simulink model "testmodel"  (R2017b)
settings: Solver=ode3  StartTime=0.0  StopTime=100  FixedStep=0.001  RelTol=1e-3
undefined symbols (not defined in the file or in its folder): DiscIntNeverNeededParam
libraries: simulink_extras x2, simulink x1
settings Model: Creator=apple  LastModifiedBy=apple
settings DebuggingCC: AlgebraicLoopMsg=none

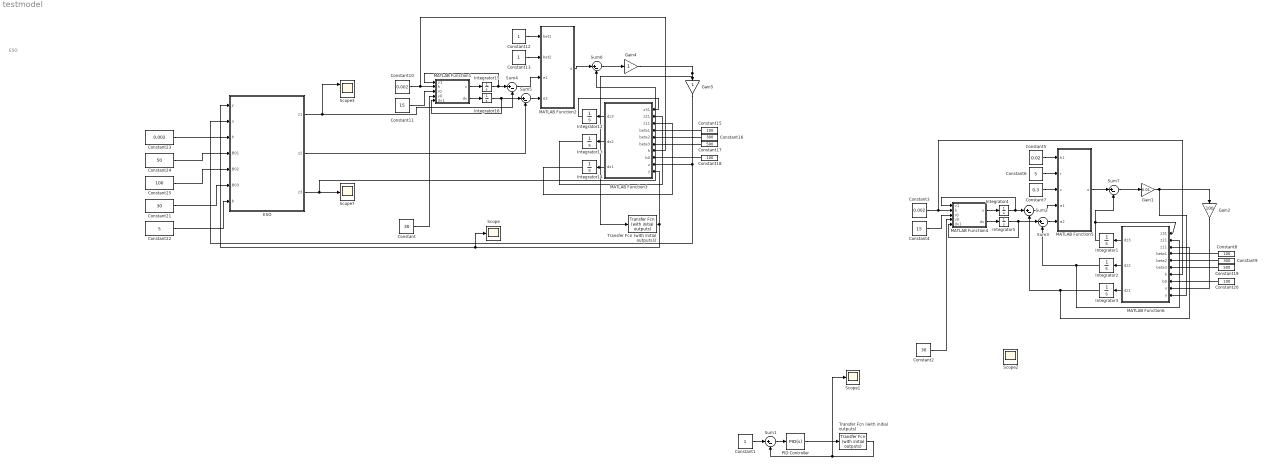
== system testmodel ==
  note: ESO
  Constant : Constant  Value=30
  Constant1 : Constant
  Constant10 : Constant  Value=0.002
  Constant11 : Constant  Value=15
  Constant12 : Constant
  Constant13 : Constant
  Constant{8,15,18,20,25} (5 alike) : Constant  Value=100
  Constant16 : Constant  Value=300
  Constant17 : Constant  Value=500
  Constant19 : Constant  Value=500
  Constant2 : Constant  Value=30
  Constant21 : Constant  Value=30
  Constant22 : Constant  Value=5
  Constant23 : Constant  Value=0.002
  Constant24 : Constant  Value=50
  Constant3 : Constant  Value=0.002
  Constant4 : Constant  Value=15
  Constant5 : Constant  Value=0.02
  Constant6 : Constant  Value=5
  Constant7 : Constant  Value=0.3
  Constant9 : Constant  Value=300
  ESO : Subsystem
  Gain1 : Gain  Gain=0.01
  Gain2 : Gain  Gain=100
  Gain4 : Gain
  Gain5 : Gain
  Integrator{1..5,12..16} (10 alike) : Integrator
  MATLAB Function1 : MATLAB Function  TreatAsAtomicUnit=on
  MATLAB Function2 : MATLAB Function  TreatAsAtomicUnit=on
  MATLAB Function3 : MATLAB Function  TreatAsAtomicUnit=on
  MATLAB Function4 : MATLAB Function  TreatAsAtomicUnit=on
  MATLAB Function5 : MATLAB Function  TreatAsAtomicUnit=on
  MATLAB Function6 : MATLAB Function  TreatAsAtomicUnit=on
  PID Controller : simulink/Continuous/PID Controller  Controller=PID  TimeDomain=Continuous-time  SampleTime=-1  IntegratorMethod=Forward Euler  FilterMethod=Forward Euler  Form=Parallel  UseFilter=on  ControllerParametersSource=internal  P=1  I=1  D=0  N=100  InitialConditionSource=internal  InitialConditionForIntegrator=0  InitialConditionForFilter=0  ExternalReset=none  LimitOutput=off  UpperSaturationLimit=inf  LowerSaturationLimit=-inf  LinearizeAsGain=on  AntiWindupMode=none  Kb=1  TrackingMode=off  Kt=1  PParamMin=[]  PParamMax=[]  IParamMin=[]  IParamMax=[]  DParamMin=[]  DParamMax=[]  NParamMin=[]  NParamMax=[]  KbParamMin=[]  KbParamMax=[]  KtParamMin=[]  KtParamMax=[]  POutMin=[]  POutMax=[]  IOutMin=[]  IOutMax=[]  DOutMin=[]  DOutMax=[]  NOutMin=[]  NOutMax=[]  KbOutMin=[]  KbOutMax=[]  KtOutMin=[]  KtOutMax=[]  IntegratorOutMin=[]  IntegratorOutMax=[]  FilterOutMin=[]  FilterOutMax=[]  SumOutMin=[]  SumOutMax=[]  SumI1OutMin=[]  SumI1OutMax=[]  SumI2OutMin=[]  SumI2OutMax=[]  SumI3OutMin=[]  SumI3OutMax=[]  SumDOutMin=[]  SumDOutMax=[]  SaturationOutMin=[]  SaturationOutMax=[]  IntegratorContinuousStateAttributes=''  IntegratorStateMustResolveToSignalObject=off  IntegratorRTWStateStorageClass=Auto  FilterContinuousStateAttributes=''  FilterStateMustResolveToSignalObject=off  FilterRTWStateStorageClass=Auto  DifferentiatorICPrevScaledInput=0  DifferentiatorOutMin=[]  DifferentiatorOutMax=[]  InitialConditionSetting=State (most efficient)  FilterDiffOutCoefMin=[]  FilterDiffOutCoefMax=[]  SumDenOutMin=[]  SumDenOutMax=[]  SumNumOutMin=[]  SumNumOutMax=[]  ReciprocalOutMin=[]  ReciprocalOutMax=[]  DivideOutMin=[]  DivideOutMax=[]  TunerSelectOption=Transfer Function Based (PID Tuner App)
  Scope{,1..2,7} (4 alike) : Scope
  Scope3 : Scope  NumInputPorts=2
  Sum{1..7} (7 alike) : Sum  Inputs=|+-
  Transfer Fcn (with initial outputs) : simulink_extras/Additional Linear/Transfer Fcn (with initial outputs)  N=[1]  D=[1 5 1]  Y0=.5  U0=0
  Transfer Fcn (with initial outputs)2 : simulink_extras/Additional Linear/Transfer Fcn (with initial outputs)  N=[1]  D=[1 5 1]  Y0=.5  U0=0
  wires:
  MATLAB Function2/1(u) -> Sum6/1
  Sum6/1 -> Gain4/1
  Gain4/1 -> Transfer Fcn (with initial outputs)2/1, Gain5/1
  Gain5/1 -> ESO/2(u), MATLAB Function3/9(u)
  Constant10/1 -> MATLAB Function3/7(h), MATLAB Function1/2(h)
  Constant11/1 -> MATLAB Function1/3(r0)
  Constant12/1 -> MATLAB Function2/1(bet1)
  Sum5/1 -> MATLAB Function2/4(e2)
  Constant13/1 -> MATLAB Function2/2(bet2)
  Sum4/1 -> MATLAB Function2/3(e1)
  Constant15/1 -> MATLAB Function3/4(beta1)
  Constant16/1 -> MATLAB Function3/5(beta2)
  Constant17/1 -> MATLAB Function3/6(beta3)
  Constant18/1 -> MATLAB Function3/8(b0)
  Constant/1 -> MATLAB Function1/4(v0)
  MATLAB Function3/1(dz3) -> Integrator12/1
  MATLAB Function3/2(dz2) -> Integrator13/1
  Integrator13/1 -> MATLAB Function3/2(z21)
  MATLAB Function3/3(dz1) -> Integrator14/1
  Integrator14/1 -> MATLAB Function3/3(z11)
  MATLAB Function1/2(dv) -> Integrator16/1
  MATLAB Function1/1(v) -> Integrator15/1
  Integrator16/1 -> MATLAB Function1/5(dv1), Sum5/1
  Integrator15/1 -> MATLAB Function1/1(v1), Sum4/1
  Constant1/1 -> Sum1/1
  Sum1/1 -> PID Controller/1
  PID Controller/1 -> Transfer Fcn (with initial outputs)/1
  Transfer Fcn (with initial outputs)/1 -> Scope1/1, Sum1/2
  Transfer Fcn (with initial outputs)2/1 -> ESO/1(y), Scope/1, MATLAB Function3/10(y)
  Integrator2/1 -> MATLAB Function6/2(z21), Sum3/2
  Constant20/1 -> MATLAB Function6/8(b0)
  Constant2/1 -> MATLAB Function4/4(v0)
  Integrator3/1 -> MATLAB Function6/3(z11), Sum2/2
  MATLAB Function4/2(dv) -> Integrator5/1
  MATLAB Function6/2(dz2) -> Integrator2/1
  Gain1/1 -> MATLAB Function6/10(y), Gain2/1
  Constant4/1 -> MATLAB Function4/3(r0)
  Sum2/1 -> MATLAB Function5/4(e1)
  Integrator1/1 -> MATLAB Function6/1(z31), Sum7/2
  MATLAB Function4/1(v) -> Integrator4/1
  Integrator4/1 -> MATLAB Function4/1(v1), Sum2/1
  Gain2/1 -> MATLAB Function6/9(u)
  Integrator5/1 -> MATLAB Function4/5(dv1), Sum3/1
  Constant6/1 -> MATLAB Function5/2(r)
  Constant3/1 -> MATLAB Function6/7(h), MATLAB Function4/2(h)
  Constant5/1 -> MATLAB Function5/1(h1)
  Sum3/1 -> MATLAB Function5/5(e2)
  Constant7/1 -> MATLAB Function5/3(c)
  Constant8/1 -> MATLAB Function6/4(beta1)
  Constant19/1 -> MATLAB Function6/6(beta3)
  Constant9/1 -> MATLAB Function6/5(beta2)
  MATLAB Function6/1(dz3) -> Integrator1/1
  MATLAB Function6/3(dz1) -> Integrator3/1
  Sum7/1 -> Gain1/1
  MATLAB Function5/1(u) -> Sum7/1
  Integrator12/1 -> MATLAB Function3/1(z31)
  ? -> Scope2/1
  ESO/1(z1) -> Sum4/2, Scope3/1
  Constant21/1 -> ESO/6(B03)
  Constant25/1 -> ESO/5(B02)
  Constant22/1 -> ESO/7(b)
  Constant23/1 -> ESO/3(h)
  ESO/3(z3) -> Sum6/2, Scope7/1
  Constant24/1 -> ESO/4(B01)
  ESO/2(z2) -> Sum5/2

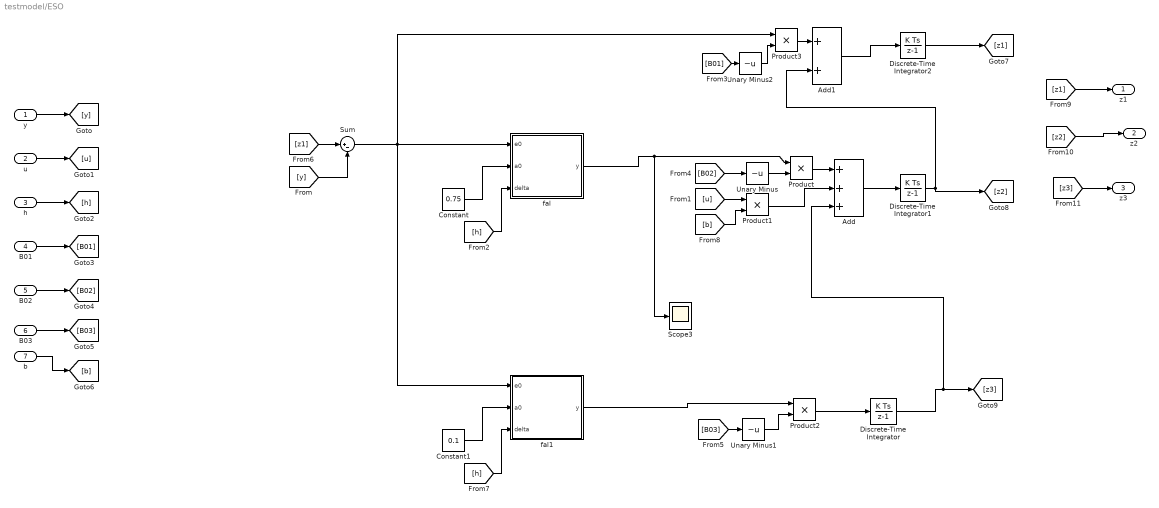
== system testmodel/ESO ==
  y : Inport
  u : Inport  Port=2
  h : Inport  Port=3
  B01 : Inport  Port=4
  B02 : Inport  Port=5
  B03 : Inport  Port=6
  b : Inport  Port=7
  Add : Sum  Inputs=+++
  Add1 : Sum
  Constant : Constant  Value=0.75
  Constant1 : Constant  Value=0.1
  Discrete-Time Integrator : DiscreteIntegrator  InitialConditionSetting=State (most efficient)  SampleTime=-1  ICPrevOutput=DiscIntNeverNeededParam  ICPrevScaledInput=DiscIntNeverNeededParam
  Discrete-Time Integrator1 : DiscreteIntegrator  InitialConditionSetting=State (most efficient)  SampleTime=-1  ICPrevOutput=DiscIntNeverNeededParam  ICPrevScaledInput=DiscIntNeverNeededParam
  Discrete-Time Integrator2 : DiscreteIntegrator  InitialConditionSetting=State (most efficient)  SampleTime=-1  ICPrevOutput=DiscIntNeverNeededParam  ICPrevScaledInput=DiscIntNeverNeededParam
  Product{,1..3} (4 alike) : Product
  Scope3 : Scope
  Sum : Sum  Inputs=|+-
  Unary Minus : UnaryMinus
  Unary Minus1 : UnaryMinus
  Unary Minus2 : UnaryMinus
  fal : MATLAB Function  TreatAsAtomicUnit=on
  fal1 : MATLAB Function  TreatAsAtomicUnit=on
  z1 : Outport
  z2 : Outport  Port=2
  z3 : Outport  Port=3
  wires:
  y/1 -> [y]
  u/1 -> [u]
  h/1 -> [h]
  B01/1 -> [B01]
  B02/1 -> [B02]
  B03/1 -> [B03]
  [h] -> fal/3(delta)
  [z1] -> Sum/1
  [y] -> Sum/2
  Constant/1 -> fal/2(a0)
  Constant1/1 -> fal1/2(a0)
  [h] -> fal1/3(delta)
  b/1 -> [b]
  [B02] -> Unary Minus/1
  Unary Minus/1 -> Product/2
  [u] -> Product1/1
  [b] -> Product1/2
  Product1/1 -> Add/2
  Product/1 -> Add/1
  fal/1(y) -> Scope3/1, Product/1
  [B03] -> Unary Minus1/1
  Unary Minus1/1 -> Product2/2
  fal1/1(y) -> Product2/1
  [B01] -> Unary Minus2/1
  Sum/1 -> Product3/1, fal1/1(e0), fal/1(e0)
  Unary Minus2/1 -> Product3/2
  Product2/1 -> Discrete-Time Integrator/1
  Add/1 -> Discrete-Time Integrator1/1
  Discrete-Time Integrator2/1 -> [z1]
  Discrete-Time Integrator1/1 -> Add1/2, [z2]
  Discrete-Time Integrator/1 -> Add/3, [z3]
  Product3/1 -> Add1/1
  Add1/1 -> Discrete-Time Integrator2/1
  [z1] -> z1/1
  [z2] -> z2/1
  [z3] -> z3/1

== matlab function testmodel/MATLAB Function1 ==
  data: v1 input; h input; r0 input; v0 input; dv1 input; v output; dv output
function [v,dv] = td(v1,h,r0,v0,dv1)

%fh = fhan(v1 - v0,dv1,r0,h)
d = r0 * h * h;
a0 = h * dv1;
y = v1 - v0 + a0;
a1 = sqrt(d * (d + 8 * abs(y)));
a2 = a0 + sign(y) * (a1 - d)/2;
a = (a0 + y -a2) * (sign(y + d) - sign(y - d))/2 + a2;
fh = -r0 * (a/d - sign(a)) * (sign(a + d) - sign(a - d))/2 - r0 * sign(a);

v = dv1;
dv = fh;
%v = v1 + h * dv1;
%dv = dv1 + h * fh;
end

== matlab function testmodel/MATLAB Function4 ==
  data: v1 input; h input; r0 input; v0 input; dv1 input; v output; dv output
function [v,dv] = td(v1,h,r0,v0,dv1)

%fh = fhan(v1 - v0,dv1,r0,h)
d = r0 * h * h;
a0 = h * dv1;
y = v1 - v0 + a0;
a1 = sqrt(d * (d + 8 * abs(y)));
a2 = a0 + sign(y) * (a1 - d)/2;
a = (a0 + y -a2) * (sign(y + d) - sign(y - d))/2 + a2;
fh = -r0 * (a/d - sign(a)) * (sign(a + d) - sign(a - d))/2 - r0 * sign(a);

v = dv1;
dv = fh;
%v = v1 + h * dv1;
%dv = dv1 + h * fh;
end

== matlab function testmodel/MATLAB Function2 ==
  data: bet1 input; bet2 input; e1 input; u output; e2 input
function u = nlsef(bet1,bet2,e1,e2)

a1 = 0.5;
a2 = 0.5;
delta1 = 0.01;
delta2 = 0.01;
u = bet1 * fal(e1,a1,delta1) + bet2 * fal(e2,a2,delta2);
end

function fe = fal(error,pow,threshold)
if abs(error) > threshold
    fe = (abs(error))^pow * sign(error);
else
    fe = error * threshold^(pow - 1);
end
end

== matlab function testmodel/MATLAB Function3 ==
  data: dz3 output; dz2 output; z31 input; z21 input; z11 input; beta1 input; beta2 input; beta3 input; h input; b0 input; dz1 output; u input; y input
function [dz3,dz2,dz1] = eso(z31,z21,z11,beta1,beta2,beta3,h,b0,u,y)

%ts = 0.001;
e = z11 - y;
dz1 = z21 - beta1 * e;
dz2 = z31 - beta2 * fal(e,0.5,h) + b0 * u;
dz3 = -beta3 * fal(e,0.25,h);

end

function fe = fal(error,pow,threshold)
if abs(error) > threshold
    fe = (abs(error))^pow * sign(error);
else
    fe = error * threshold^(pow - 1);
end
end

== matlab function testmodel/MATLAB Function5 ==
  data: h1 input; r input; c input; e1 input; u output; e2 input
function u = nlsef(h1,r,c,e1,e2)

%fh = fhan(e1,c * e2,r,h1)
d = r * h1 * h1;
a0 = h1 * c * e2;
y = e1 + a0;
a1 = sqrt(d * (d + 8 * abs(y)));
a2 = a0 + sign(y) * (a1 - d)/2;
a = (a0 + y -a2) * (sign(y + d) - sign(y - d))/2 + a2;
fh = -r * (a/d - sign(a)) * (sign(a + d) - sign(a - d))/2 - r * sign(a);
u = fh;
end

== matlab function testmodel/MATLAB Function6 ==
  data: dz3 output; dz2 output; z31 input; z21 input; z11 input; beta1 input; beta2 input; beta3 input; h input; b0 input; dz1 output; u input; y input
function [dz3,dz2,dz1] = eso(z31,z21,z11,beta1,beta2,beta3,h,b0,u,y)

%ts = 0.001;
e = z11 - y;
dz1 = z21 - beta1 * e;
dz2 = z31 - beta2 * fal(e,0.5,h) + b0 * u;
dz3 = -beta3 * fal(e,0.25,h);

end

function fe = fal(error,pow,threshold)
if abs(error) > threshold
    fe = (abs(error))^pow * sign(error);
else
    fe = error * threshold^(pow - 1);
end
end

== matlab function testmodel/ESO/fal ==
  data: e0 input; y output; a0 input; delta input
function y = fcn(e0,a0,delta)
if(abs(e0)>delta)
    y=((abs(e0))^a0)*sign(e0);
else
    y=e0/(delta^(1-a0));
end

== matlab function testmodel/ESO/fal1 ==
  data: e0 input; y output; a0 input; delta input
function y = fcn(e0,a0,delta)
if(abs(e0)>delta)
    y=(abs(e0))^a0*sign(e0);
else
    y=e0/(delta^(1-a0));
end
